simulink model "system_sim_v2_test1"  (R2015a)
settings: Solver=ode45  StartTime=0.0  StopTime=3600*4  FixedStep=0.05  RelTol=1e-3
values from neighbouring files (symbols this model uses):
  area = 1.2    [run_sim_auto.m]    (also in run_sim_test4.m = 2; sim_testing.m; wrkspc_no_1.mat; wrkspc_no_10.mat)
  Cd = 0.6    [run_sim_auto.m]    (also in run_sim_test4.m = 1; sim_testing.m; wrkspc_no_1.mat; wrkspc_no_10.mat)
  Crr = 0.005    [run_sim_test4.m]    (also in wrkspc_no_1.mat; wrkspc_no_10.mat; wrkspc_no_18.mat; wrkspc_no_22.mat)
  end_x = x_in_m(length(x_in_m))    [run_sim_auto.m]    (also in run_sim_v2.m; wrkspc_no_1.mat = 44100; wrkspc_no_10.mat = 48084; wrkspc_no_18.mat = 8912)
  fmax = max_moving_force    [run_sim_auto.m]    (also in run_sim_v2.m; wrkspc_no_1.mat = 666.666666667; wrkspc_no_10.mat = 666.666666667; wrkspc_no_18.mat = 666.666666667)
  g = 9.81    [run_sim.m]    (also in run_sim_auto.m; run_sim_test.m; run_sim_test4.m; run_sim_v2.m)
  Kp = 700    [run_sim_auto.m]    (also in run_sim_v2.m = 150; sim_testing.m; wrkspc_no_1.mat; wrkspc_no_10.mat)
  m = 210    [run_sim_auto.m]    (also in run_sim_test4.m = 150; sim_testing.m; wrkspc_no_1.mat; wrkspc_no_10.mat)
  max_brake_force = brake_force    [run_sim_auto.m]    (also in run_sim_v2.m; wrkspc_no_1.mat = 1000; wrkspc_no_10.mat = 1000; wrkspc_no_18.mat = 1000)
  rho_air = 1.225    [run_sim.m]    (also in run_sim_auto.m; run_sim_test.m; run_sim_test4.m; run_sim_v2.m)
  target_speed_m_s = 4.16    [run_sim_test4.m]    (also in wrkspc_no_1.mat = 4.16666666667; wrkspc_no_10.mat = 4.16666666667; wrkspc_no_18.mat = 4.16666666667; wrkspc_no_22.mat = 4.16666666667)
settings Model: Creator=marco  LastModifiedBy=marco

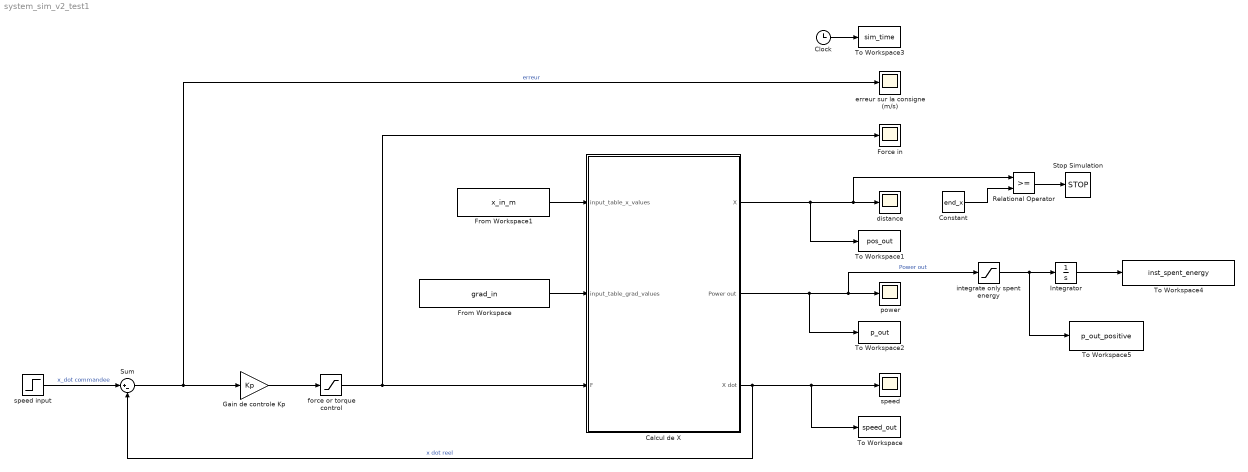
== system system_sim_v2_test1 ==
  Calcul de X : Subsystem
  Clock : Clock
  Constant : Constant  Value=end_x
  Force in : Scope
      settings: TimeRange=60  YMin=4  YMax=5.5  SaveName=ScopeData5  MaxDataPoints=scope_history
  From Workspace : FromWorkspace  VariableName=grad_in  SampleTime=0
  From Workspace1 : FromWorkspace  VariableName=x_in_m  SampleTime=0
  Gain de controle Kp : Gain  Gain=Kp
  Integrator : Integrator
  Relational Operator : RelationalOperator  OutDataTypeStr=boolean
  Stop Simulation : Stop
  Sum : Sum  Inputs=|+-
  To Workspace : ToWorkspace  VariableName=speed_out  SampleTime=-1
      settings: Save2DSignal=2-D array (concatenate along first dimension)
  To Workspace1 : ToWorkspace  VariableName=pos_out  SampleTime=-1
      settings: Save2DSignal=2-D array (concatenate along first dimension)
  To Workspace2 : ToWorkspace  VariableName=p_out  SampleTime=-1
      settings: Save2DSignal=2-D array (concatenate along first dimension)
  To Workspace3 : ToWorkspace  VariableName=sim_time  SampleTime=-1
      settings: Save2DSignal=2-D array (concatenate along first dimension)
  To Workspace4 : ToWorkspace  VariableName=inst_spent_energy  SampleTime=-1
      settings: Save2DSignal=2-D array (concatenate along first dimension)
  To Workspace5 : ToWorkspace  VariableName=p_out_positive  SampleTime=-1
      settings: Save2DSignal=2-D array (concatenate along first dimension)
  distance : Scope
      settings: MaxDataPoints=scope_history
  erreur sur la consigne (m/s) : Scope
      settings: SaveName=ScopeData6  MaxDataPoints=scope_history
  force or torque control : Saturate  UpperLimit=fmax  LowerLimit=-max_brake_force
  integrate only spent energy : Saturate  UpperLimit=fmax*target_speed_m_s*2  LowerLimit=0
  power : Scope
      settings: TimeRange=700  YMin=-200  YMax=700  SaveName=ScopeData4  MaxDataPoints=scope_history
  speed : Scope
      settings: MaxDataPoints=scope_history
  speed input : Step  Time=0.1  After=target_speed_m_s  SampleTime=1
  wires:
  speed input/1 -> Sum/1  "x_dot commandee"
  From Workspace1/1 -> Calcul de X/1(input_table_x_values)
  From Workspace/1 -> Calcul de X/2(input_table_grad_values)
  Sum/1 -> Gain de controle Kp/1, erreur sur la consigne (m/s)/1  "erreur"
  Gain de controle Kp/1 -> force or torque control/1
  force or torque control/1 -> Calcul de X/3(F), Force in/1
  Calcul de X/3(X dot) -> To Workspace/1, speed/1, Sum/2  "x dot reel"
  Calcul de X/2(Power out) -> To Workspace2/1, integrate only spent energy/1, power/1  "Power out"
  Calcul de X/1(X) -> To Workspace1/1, Relational Operator/1, distance/1
  Constant/1 -> Relational Operator/2
  Relational Operator/1 -> Stop Simulation/1
  Clock/1 -> To Workspace3/1
  Integrator/1 -> To Workspace4/1
  integrate only spent energy/1 -> To Workspace5/1, Integrator/1

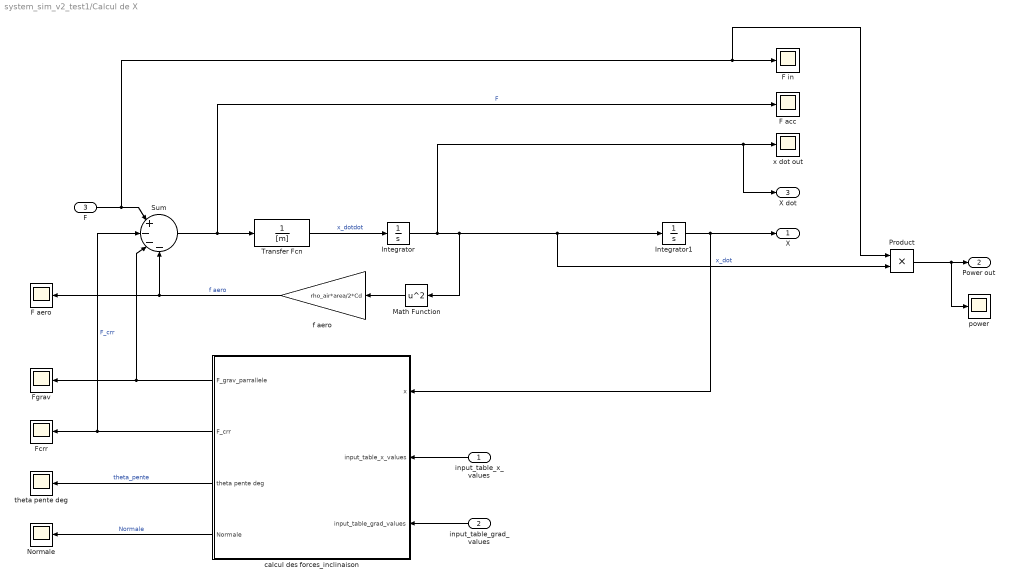
== system system_sim_v2_test1/Calcul de X ==
  input_table_x_values : Inport
  input_table_grad_values : Inport  Port=2
  F : Inport  Port=3
  F acc : Scope
      settings: YMin=-1398.32  YMax=-1398.12  SaveName=ScopeData7  MaxDataPoints=scope_history
  F aero : Scope
      settings: SaveName=ScopeData14  MaxDataPoints=scope_history
  F in : Scope
      settings: SaveName=ScopeData12  MaxDataPoints=scope_history  SampleTime=1
  Fcrr : Scope
      settings: SaveName=ScopeData10  MaxDataPoints=scope_history
  Fgrav : Scope
      settings: SaveName=ScopeData9  MaxDataPoints=scope_history
  Integrator : Integrator
  Integrator1 : Integrator
  Math Function : Math  Operator=square  SaturateOnIntegerOverflow=on
  Normale : Scope
      settings: SaveName=ScopeData2  MaxDataPoints=scope_history
  Product : Product
  Sum : Sum  Inputs=|+---
  Transfer Fcn : TransferFcn  Denominator=[m]
  calcul des forces_inclinaison : Subsystem
  f aero : Gain  Gain=rho_air*area/2*Cd
  power : Scope
      settings: SaveName=ScopeData11  MaxDataPoints=scope_history
  "theta pente deg " : Scope
      settings: SaveName=ScopeData3  MaxDataPoints=scope_history
  x dot out : Scope
      settings: SaveName=ScopeData13  MaxDataPoints=scope_history
  X : Outport
  Power out : Outport  Port=2
  X dot : Outport  Port=3
  wires:
  Sum/1 -> F acc/1, Transfer Fcn/1  "F"
  Transfer Fcn/1 -> Integrator/1  "x_dotdot"
  Integrator/1 -> X dot/1, x dot out/1, Math Function/1, Product/2, Integrator1/1  "x_dot"
  f aero/1 -> F aero/1, Sum/4  "f aero"
  input_table_x_values/1 -> calcul des forces_inclinaison/2(input_table_x_values)
  input_table_grad_values/1 -> calcul des forces_inclinaison/3(input_table_grad_values)
  Math Function/1 -> f aero/1
  Integrator1/1 -> calcul des forces_inclinaison/1(x), X/1
  calcul des forces_inclinaison/3(theta pente deg) -> "theta pente deg "/1  "theta_pente"
  calcul des forces_inclinaison/2(F_crr) -> Sum/2, Fcrr/1  "F_crr"
  calcul des forces_inclinaison/1(F_grav_parrallele) -> Sum/3, Fgrav/1
  calcul des forces_inclinaison/4(Normale) -> Normale/1  "Normale"
  F/1 -> Product/1, F in/1, Sum/1
  Product/1 -> power/1, Power out/1

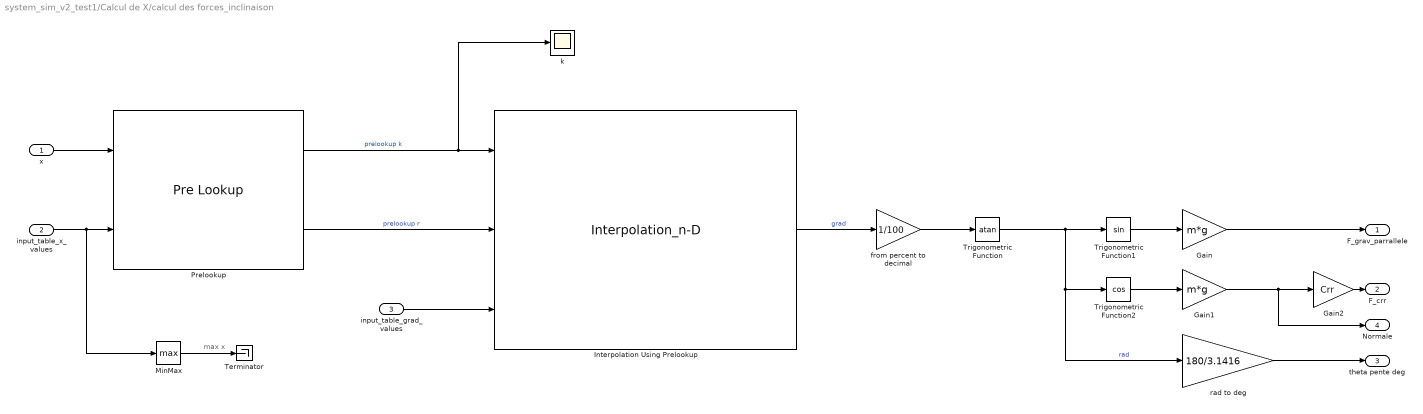
== system system_sim_v2_test1/Calcul de X/calcul des forces_inclinaison ==
  note: max x
  x : Inport
  input_table_x_values : Inport  Port=2
  input_table_grad_values : Inport  Port=3
  Gain : Gain  Gain=m*g
  Gain1 : Gain  Gain=m*g
  Gain2 : Gain  Gain=Crr
  Interpolation Using Prelookup : Interpolation_n-D  NumberOfTableDimensions=1  TableSource=Input port  InternalRulePriority=Speed
      settings: InputPortMap=u0,u1,p2
  MinMax : MinMax  Function=max
  Prelookup : PreLookup  BreakpointsDataSource=Input port  BreakpointsData=[10:10:110]  ExtrapMethod=Linear
      settings: InputPortMap=u0,p1
  Terminator : Terminator
  Trigonometric Function : Trigonometry  Operator=atan
  Trigonometric Function1 : Trigonometry
  Trigonometric Function2 : Trigonometry  Operator=cos
  from percent to decimal : Gain  Gain=1/100
  k : Scope
      settings: SaveName=ScopeData8  MaxDataPoints=scope_history
  rad to deg : Gain  Gain=180/3.1416
  F_grav_parrallele : Outport
  F_crr : Outport  Port=2
  theta pente deg : Outport  Port=3
  Normale : Outport  Port=4
  wires:
  x/1 -> Prelookup/1
  Interpolation Using Prelookup/1 -> from percent to decimal/1  "grad"
  Trigonometric Function1/1 -> Gain/1
  Trigonometric Function2/1 -> Gain1/1
  Gain1/1 -> Normale/1, Gain2/1
  Prelookup/1 -> k/1, Interpolation Using Prelookup/1  "prelookup k"
  Prelookup/2 -> Interpolation Using Prelookup/2  "prelookup r"
  input_table_grad_values/1 -> Interpolation Using Prelookup/3
  Trigonometric Function/1 -> rad to deg/1, Trigonometric Function2/1, Trigonometric Function1/1  "rad"
  from percent to decimal/1 -> Trigonometric Function/1
  input_table_x_values/1 -> MinMax/1, Prelookup/2
  Gain/1 -> F_grav_parrallele/1
  Gain2/1 -> F_crr/1
  rad to deg/1 -> theta pente deg/1
  MinMax/1 -> Terminator/1
